simulink model "mass_spring_damper_simulink_model"  (R2024b)
settings: Solver=VariableStepAuto  StartTime=0.0  StopTime=10.0  RelTol=1e-3
undefined symbols (not defined in the file): b, f, k, M
settings Model: Creator=Lenovo  LastModifiedBy=Lenovo

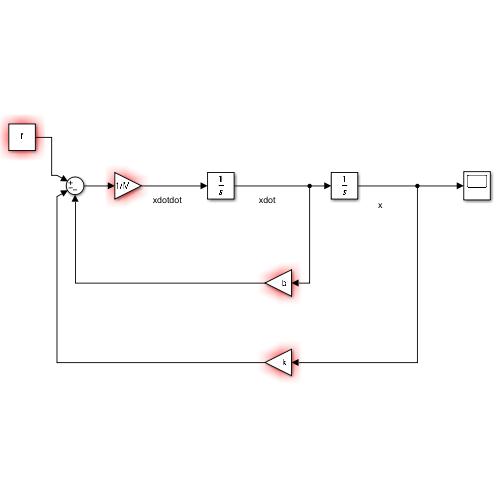
[thumbnail: Simulink's stored preview of the top-level diagram]
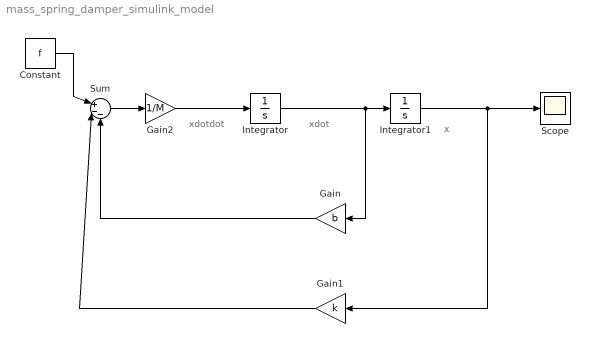
== system mass_spring_damper_simulink_model ==
  note: xdotdot
  note: xdot
  note: x
  Constant : Constant  Value=f
  Gain : Gain  Gain=b
  Gain1 : Gain  Gain=k
  Gain2 : Gain  Gain=1/M
  Integrator : Integrator
  Integrator1 : Integrator
  Scope : Scope
  Sum : Sum  Inputs=|+--
  wires:
  Integrator/1 -> Gain/1, Integrator1/1
  Integrator1/1 -> Gain1/1, Scope/1
  Gain2/1 -> Integrator/1
  Sum/1 -> Gain2/1
  Constant/1 -> Sum/1
  Gain/1 -> Sum/3
  Gain1/1 -> Sum/2
